simulink model "OhmicResistance"  (R2012b)
settings: Solver=ode45  StartTime=0.0  StopTime=10.0  RelTol=1e-3
settings Model: Creator=sz609516  LastModifiedBy=sz609516
settings DataIOCC: SignalLoggingSaveFormat=ModelDataLogs
settings DebuggingCC: FcnCallInpInsideContextMsg=EnableAllAsWarning
settings GRTTargetCC: CombineOutputUpdateFcns=off  GRTInterface=on

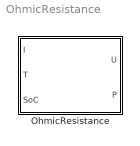
== system OhmicResistance ==
  OhmicResistance : Subsystem

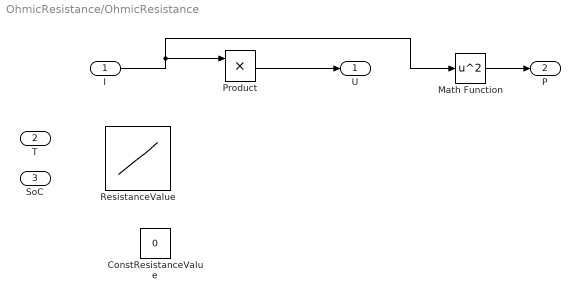
== system OhmicResistance/OhmicResistance ==
  I : Inport
  T : Inport  Port=2
  SoC : Inport  Port=3
  ConstResistanceValue : Constant  Value=0
  Math Function : Math  Operator=square  SaturateOnIntegerOverflow=on
  Product : Product  RndMeth=Zero
  ResistanceValue : Lookup_n-D  Table=[1,2,3;4,5,6;7,8,9]  ExtrapMethod=Clip  RndMeth=Simplest  InputSameDT=on
  U : Outport
  P : Outport  Port=2
  wires:
  Product/1 -> U/1
  I/1 -> Product/1, Math Function/1
  Math Function/1 -> P/1
